simulink model "Model_Rover"  (R2024b)
settings: Solver=VariableStepAuto  StartTime=0.0  StopTime=30  MaxStep=0.1  RelTol=1e-3
InitFcn:
  | main
values from neighbouring files (symbols this model uses):
  rad_b = 0.025    [main.m]    (also in main_2.0.m; main_3.0.m)
  rad_l = 0.05    [main.m]    (also in main_2.0.m; main_3.0.m)
  rover_radr = 0.05    [main.m]    (also in main_2.0.m; main_3.0.m)
  roverb = 0.3    [main.m]    (also in main_2.0.m = 0.2; main_3.0.m)
  roverh = 0.2    [main.m]    (also in main_2.0.m; main_3.0.m)
  roverl = 0.4    [main.m]    (also in main_2.0.m = 0.1; main_3.0.m; plotdata.mat = 0.5)
  sp = [0, 0]    [main.m]    (also in main_2.0.m = [1,1]; main_3.0.m; plotdata.mat = [0 0])
  x_pfad = pos(1)    [pfadplaner.m]    (also in pfadplaner_2.0.m)
  X_sp = sp(1)    [main_2.0.m]
  y_pfad = pos(2)    [pfadplaner.m]    (also in pfadplaner_2.0.m)
  Y_sp = sp(2)    [main_2.0.m]
settings Model: Creator=thiagothielecke  LastModifiedBy=melis

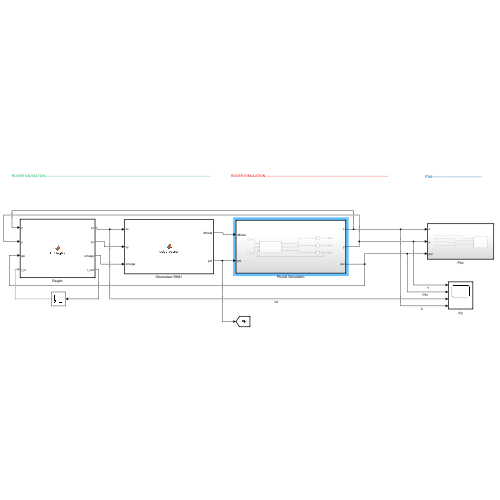
[thumbnail: Simulink's stored preview of the top-level diagram]
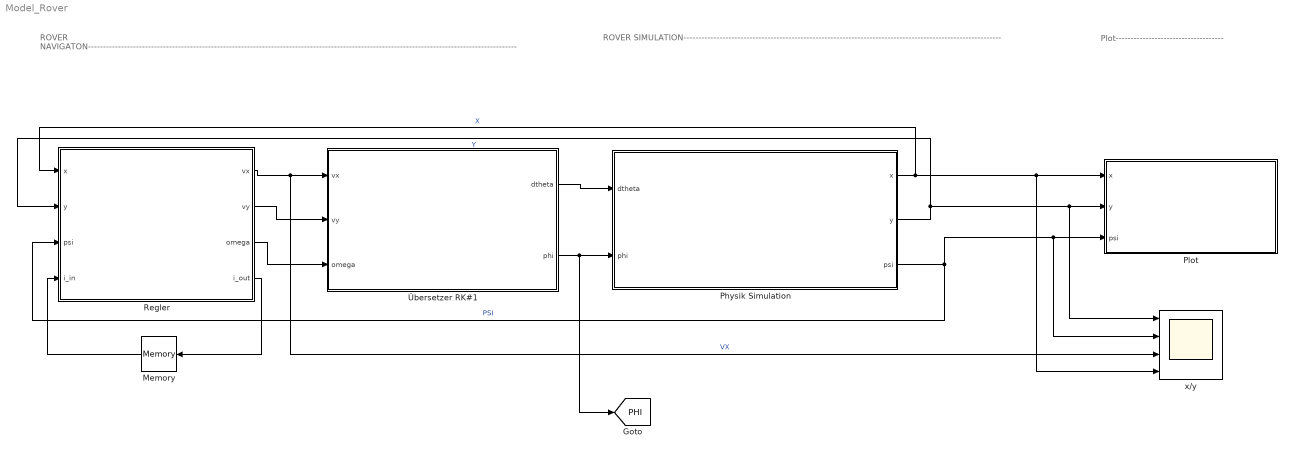
== system Model_Rover ==
  note: Plot------------------------------------
  note: ROVER SIMULATION----------------------------------------------------------------------------------------------------------
  note: ROVER NAVIGATON-----------------------------------------------------------------------------------------------------------------------------------------------
  Memory : Memory  InitialCondition=1  InheritSampleTime=on
  Physik Simulation : Subsystem
  Plot : Subsystem
  Regler : MATLAB Function  TreatAsAtomicUnit=on
  x/y : Scope  NumInputPorts=4
  Übersetzer RK#1 : MATLAB Function  TreatAsAtomicUnit=on
  tag scope: PHI=global
  wires:
  Übersetzer RK#1/2(phi) -> [PHI], Physik Simulation/2(phi)
  Übersetzer RK#1/1(dtheta) -> Physik Simulation/1(dtheta)
  Regler/3(omega) -> Übersetzer RK#1/3(omega)
  Physik Simulation/1(x) -> Regler/1(x), x/y/4, Plot/1(x)  "X"
  Physik Simulation/2(y) -> Regler/2(y), x/y/1, Plot/2(y)  "Y"
  Physik Simulation/3(psi) -> x/y/2, Plot/3(psi), Regler/3(psi)  "PSI"
  Regler/2(vy) -> Übersetzer RK#1/2(vy)
  Memory/1 -> Regler/4(i_in)
  Regler/4(i_out) -> Memory/1
  Regler/1(vx) -> x/y/3, Übersetzer RK#1/1(vx)  "VX"

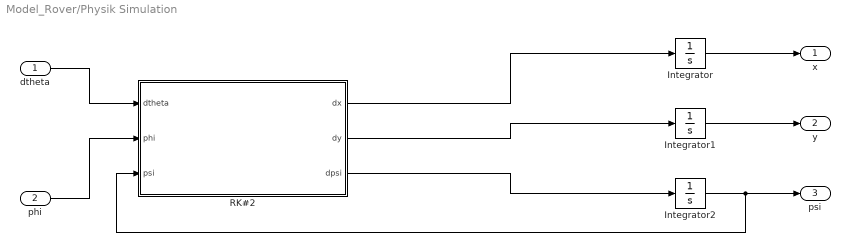
== system Model_Rover/Physik Simulation ==
  dtheta : Inport
  phi : Inport  Port=2
  Integrator : Integrator  InitialCondition=sp(1)
  Integrator1 : Integrator  InitialCondition=sp(2)
  Integrator2 : Integrator
  RK#2 : MATLAB Function  TreatAsAtomicUnit=on
  x : Outport
  y : Outport  Port=2
  psi : Outport  Port=3
  wires:
  Integrator2/1 -> RK#2/3(psi), psi/1
  dtheta/1 -> RK#2/1(dtheta)
  phi/1 -> RK#2/2(phi)
  Integrator1/1 -> y/1
  Integrator/1 -> x/1
  RK#2/1(dx) -> Integrator/1
  RK#2/3(dpsi) -> Integrator2/1
  RK#2/2(dy) -> Integrator1/1

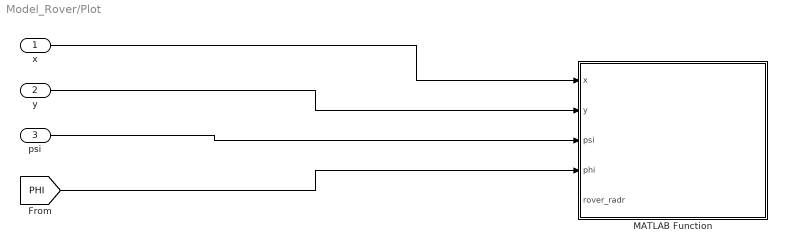
== system Model_Rover/Plot ==
  x : Inport
  y : Inport  Port=2
  psi : Inport  Port=3
  MATLAB Function : MATLAB Function  TreatAsAtomicUnit=on
  wires:
  x/1 -> MATLAB Function/1(x)
  y/1 -> MATLAB Function/2(y)
  psi/1 -> MATLAB Function/3(psi)
  [PHI] -> MATLAB Function/4(phi)

== matlab function Model_Rover/Regler ==
  settings: updateMethod=CONTINUOUS  sampleTime=[0.1 0]
  data: vx output; vy output; x input; y input; psi input; omega output; i_in input; i_out output; x_pfad parameter; y_pfad parameter
function [vx, vy, omega, i_out] = P_Regler(x, y, psi, i_in, x_pfad, y_pfad)
%#codegen

% Reglerparameter
Kp_pos    = 5.0;
Kp_phi    = 0.0;    % Kp_phi = 0 -> Drehung während Fahrt nicht berücksichtigt
tol_dist  = 0.1;
max_omega = 1.0;

% Index-Initialisierung und stellt sicher dass der Index im gültigen
% Bereich liegt
i = max(1, min(i_in, length(x_pfad)));

% Sollpunkt
x_soll = x_pfad(i);
y_soll = y_pfad(i);

% Fehlerberechnung
fehler_x = x_soll - x;
fehler_y = y_soll - y;
entfernung = sqrt(fehler_x^2 + fehler_y^2);

% Zielwinkel (optional)
winkel_zum_ziel = atan2(fehler_y, fehler_x);
fehler_phi = atan2(sin(winkel_zum_ziel - psi), cos(winkel_zum_ziel - psi));

% Wegpunkt erreicht?!->nächsten waypoint holen i++
if entfernung < tol_dist && i < length(x_pfad)
    i = i + 1;
end

% Positionsregler
vx = Kp_pos * fehler_x;
vy = Kp_pos * fehler_y;

% 
% Orientierung optional ignorieren
omega = Kp_phi * fehler_phi;
omega = max(min(omega, max_omega), -max_omega);

% Ausgabe
i_out = i;

end

== matlab function Model_Rover/Übersetzer RK#1 ==
  data: vx input; vy input; omega input; roverb parameter; dtheta output; phi output; roverl parameter; rover_radr parameter
function [dtheta, phi] = uebersetzer(vx,vy, omega, roverb, roverl, rover_radr)
%%%%%%(RK#1)%%%%%%%%%%
% Vorberechnung
b2 = roverb/2;
l2 = roverl/2;

% Lenkwinkel phi_i
phi = zeros(4,1); % erstellt Vektor 4x1 mit 0er
phi(1) = atan2(vy + omega * l2, vx + omega * b2);
phi(2) = atan2(vy + omega * l2, vx - omega * b2);
phi(3) = atan2(vy - omega * l2, vx - omega * b2);
phi(4) = atan2(vy - omega * l2, vx + omega * b2);

% Radgeschwindigkeiten theta_dot_i
dtheta = zeros(4,1);
dtheta(1) = (1/rover_radr) * sqrt((vx + omega * b2)^2 + (vy + omega * l2)^2);
dtheta(2) = (1/rover_radr) * sqrt((vx - omega * b2)^2 + (vy + omega * l2)^2);
dtheta(3) = (1/rover_radr) * sqrt((vx - omega * b2)^2 + (vy - omega * l2)^2);
dtheta(4) = (1/rover_radr) * sqrt((vx + omega * b2)^2 + (vy - omega * l2)^2);

== matlab function Model_Rover/Physik Simulation/RK#2 ==
  data: dtheta input; dx output; phi input; psi input; rover_radr parameter; roverb parameter; dy output; dpsi output; X_sp parameter; Y_sp parameter
function [dx, dy, dpsi]  = fcn(dtheta, phi, psi, rover_radr, roverb, X_sp, Y_sp)

%Initialisierung als Skalar
dx = X_sp;
dy = Y_sp;
dpsi = 0;

%Rotationsmatrix
rmatrix=[cos(psi) sin(psi) 0; -sin(psi) cos(psi) 0; 0 0 1 ];

%berechnet die translatorische und rotatorische Geschwindigkeit des Roboters im lokalen Koordinatensystem
m2 = [rover_radr/4 * (dtheta(1)*cos(phi(1)) + dtheta(2)*cos(phi(2)) + dtheta(3)*cos(phi(3)) +  dtheta(4)*cos(phi(4)));
        
      rover_radr/4 * (dtheta(1)*sin(phi(1)) + dtheta(2)*sin(phi(2)) + dtheta(3)*sin(phi(3)) +  dtheta(4)*sin(phi(4)));

      rover_radr/2*roverb * (dtheta(1)*cos(phi(1)) - dtheta(2)*cos(phi(2)) - dtheta(3)*cos(phi(3)) +  dtheta(4)*cos(phi(4))) ];


%rotiert sie in globale Koordinaten
dxdydpsi = rmatrix * m2;


dx = dxdydpsi(1);
dy = dxdydpsi(2) ;
dpsi = dxdydpsi(3);

== matlab function Model_Rover/Plot/MATLAB Function ==
  data: x input; y input; psi input; phi input; roverl parameter; roverb parameter; roverh parameter; rad_l parameter; rad_b parameter; rover_radr input
function update_visu(x, y, psi, phi, roverl, roverb, roverh, rad_l, rad_b, rover_radr)
%#codegen
coder.extrinsic('update_visu');

x = double(x);
y = double(y);
psi = double(psi);
phi = double(phi);

update_visu(x, y, psi, phi, roverl, roverb, rad_l, rad_b, rover_radr, roverh);
